simulink model "NonLinearControl"  (R2021b)
settings: Solver=VariableStepAuto  StartTime=0  StopTime=500  RelTol=1e-3
values from neighbouring files (symbols this model uses):
  accelerationLimit = 0.37    [ltdSimulationParameters.m]
  ageTrain = 0.85    [ltdSimulationParameters.m]
  decelerationLimit = 1.18    [ltdSimulationParameters.m]
  K = place(A,B,pole)    [ltdSimulationParameters.m]
  Ka = 0.07    [ltdSimulationParameters.m]
  M = 54.5    [ltdSimulationParameters.m]
  m = M * 10^3 + (load * weight)    (= 58980)    [ltdSimulationParameters.m]
  nP = 6    [ltdSimulationParameters.m]
  speedLimit = 55.88    [ltdSimulationParameters.m]
  theta = 4e-4    (= 0.0004)    [ltdSimulationParameters.m]
  wP = m/nP    (= 9830)    [ltdSimulationParameters.m]
  x_1 = 0    [ltdSimulationParameters.m]
  x_2 = 0    [ltdSimulationParameters.m]
undefined symbols (not defined in the file or in its folder): displaceRequired, magnitude
settings Model: SimulationMode=rapid-accelerator  Creator=User  LastModifiedBy=User
settings SolverCC: AlgebraicLoopSolver=TrustRegion
settings DebuggingCC: SFMachineParentedDataDiag=warning

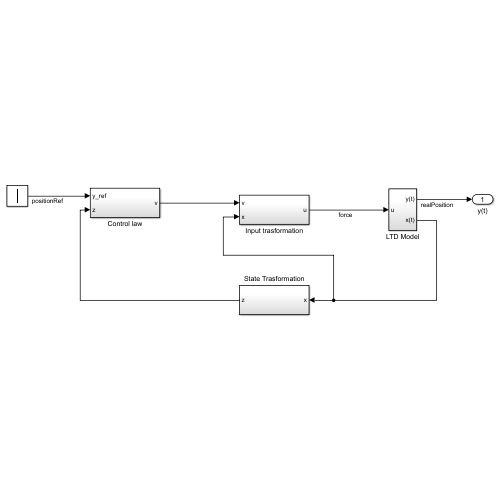
[thumbnail: Simulink's stored preview of the top-level diagram]
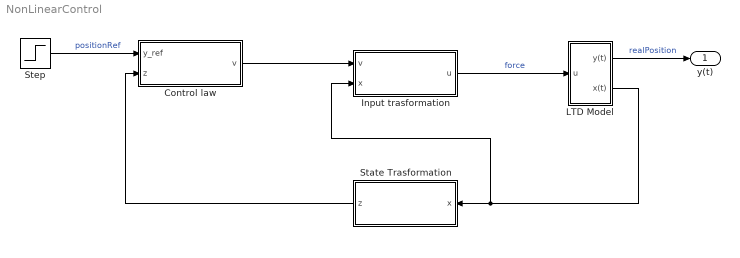
== system NonLinearControl ==
  Control law : Subsystem
  Input trasformation : Subsystem
  LTD Model : Subsystem
  State Trasformation : Subsystem
  Step : Step  After=displaceRequired  SampleTime=0
  y(t) : Outport
  wires:
  Input trasformation/1(u) -> LTD Model/1(u)  "force"
  LTD Model/2(x(t)) -> State Trasformation/1(x), Input trasformation/2(x)
  LTD Model/1(y(t)) -> y(t)/1  "realPosition"
  State Trasformation/1(z) -> Control law/2(z)
  Control law/1(v) -> Input trasformation/1(v)
  Step/1 -> Control law/1(y_ref)  "positionRef"

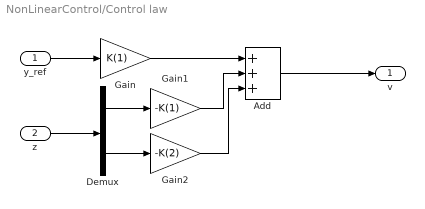
== system NonLinearControl/Control law ==
  y_ref : Inport
  z : Inport  Port=2
  Add : Sum  Inputs=+++
  Demux : Demux  Outputs=2
  Gain : Gain  Gain=K(1)
  Gain1 : Gain  Gain=-K(1)
  Gain2 : Gain  Gain=-K(2)
  v : Outport
  wires:
  z/1 -> Demux/1
  y_ref/1 -> Gain/1
  Gain/1 -> Add/1
  Demux/1 -> Gain1/1
  Demux/2 -> Gain2/1
  Gain1/1 -> Add/2
  Gain2/1 -> Add/3
  Add/1 -> v/1

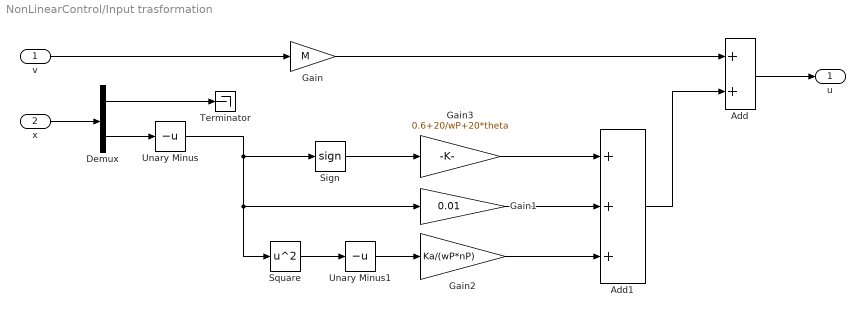
== system NonLinearControl/Input trasformation ==
  v : Inport
  x : Inport  Port=2
  Add : Sum
  Add1 : Sum  Inputs=+++
  Demux : Demux  Outputs=2
  Gain : Gain  Gain=M
  Gain1 : Gain  Gain=0.01
  Gain2 : Gain  Gain=Ka/(wP*nP)
  Gain3 : Gain  Gain=0.6+20/wP+20*theta
  Sign : Signum
  Square : Math  Operator=square  SaturateOnIntegerOverflow=on
  Terminator : Terminator
  Unary Minus : UnaryMinus
  Unary Minus1 : UnaryMinus
  u : Outport
  wires:
  v/1 -> Gain/1
  Gain/1 -> Add/1
  x/1 -> Demux/1
  Demux/1 -> Terminator/1
  Gain1/1 -> Add1/2
  Gain2/1 -> Add1/3
  Add1/1 -> Add/2
  Add/1 -> u/1
  Unary Minus1/1 -> Gain2/1
  Square/1 -> Unary Minus1/1
  Demux/2 -> Unary Minus/1
  Unary Minus/1 -> Sign/1, Gain1/1, Square/1
  Gain3/1 -> Add1/1
  Sign/1 -> Gain3/1

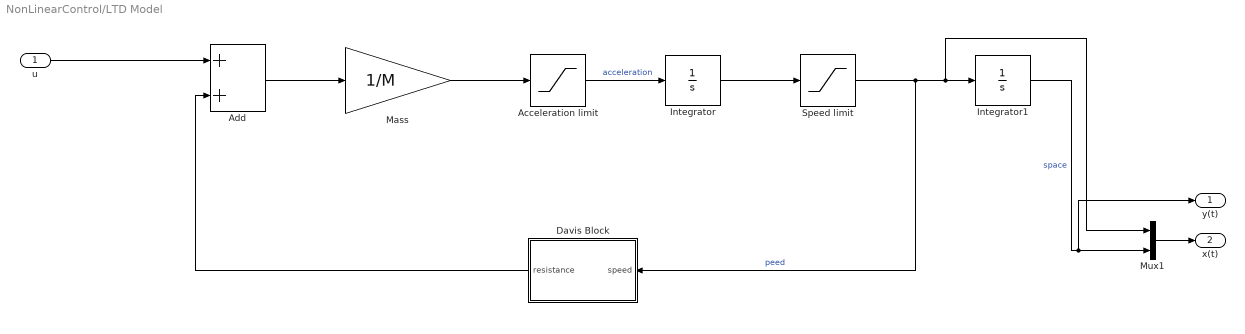
== system NonLinearControl/LTD Model ==
  u : Inport
  Acceleration limit : Saturate  UpperLimit=accelerationLimit  LowerLimit=-decelerationLimit
  Add : Sum
  Davis Block : Subsystem
  Integrator : Integrator  InitialCondition=x_2
  Integrator1 : Integrator  InitialCondition=x_1
  Mass : Gain  Gain=1/M
  Mux1 : Mux  Inputs=2
  Speed limit : Saturate  UpperLimit=speedLimit  LowerLimit=-speedLimit
  y(t) : Outport
  x(t) : Outport  Port=2
  wires:
  Acceleration limit/1 -> Integrator/1  "acceleration"
  Mass/1 -> Acceleration limit/1
  Speed limit/1 -> Davis Block/1(speed), Mux1/1, Integrator1/1  "peed"
  Integrator1/1 -> Mux1/2, y(t)/1  "space"
  Mux1/1 -> x(t)/1
  Integrator/1 -> Speed limit/1
  Add/1 -> Mass/1
  u/1 -> Add/1
  Davis Block/1(resistance) -> Add/2

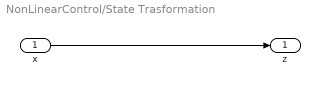
== system NonLinearControl/State Trasformation ==
  x : Inport
  z : Outport
  wires:
  x/1 -> z/1

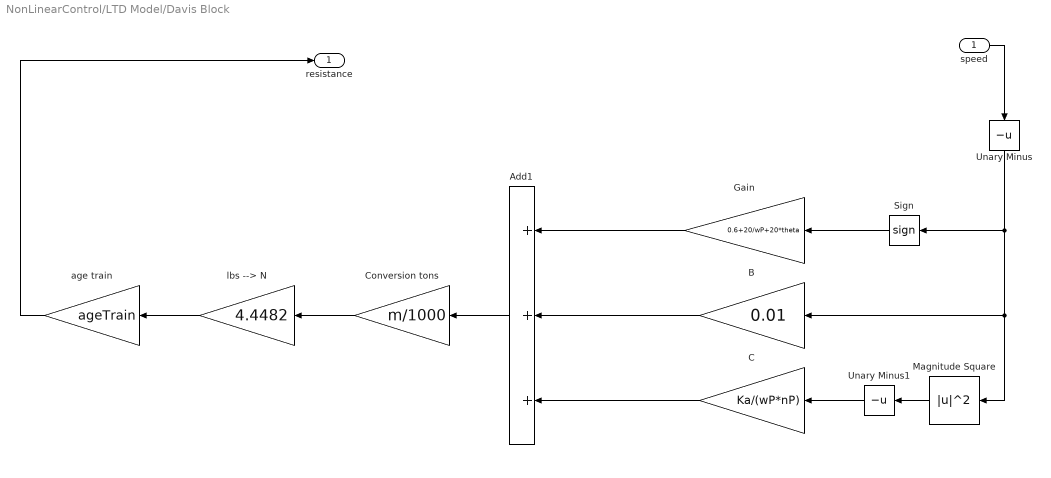
== system NonLinearControl/LTD Model/Davis Block ==
  speed : Inport
  Add1 : Sum  Inputs=+++
  B : Gain  Gain=0.01
  C : Gain  Gain=Ka/(wP*nP)
  Conversion tons : Gain  Gain=m/1000
  Gain : Gain  Gain=0.6+20/wP+20*theta
  Magnitude Square : Math  Operator=magnitude^2  SignedPower=on  RndMeth=Zero  SaturateOnIntegerOverflow=on
  Sign : Signum
  Unary Minus : UnaryMinus
  Unary Minus1 : UnaryMinus
  age train : Gain  Gain=ageTrain
  lbs --> N : Gain  Gain=4.4482
  resistance : Outport
  wires:
  lbs --> N/1 -> age train/1
  Unary Minus/1 -> Magnitude Square/1, B/1, Sign/1
  Gain/1 -> Add1/1
  Magnitude Square/1 -> Unary Minus1/1
  Conversion tons/1 -> lbs --> N/1
  Add1/1 -> Conversion tons/1
  B/1 -> Add1/2
  C/1 -> Add1/3
  Unary Minus1/1 -> C/1
  speed/1 -> Unary Minus/1
  Sign/1 -> Gain/1
  age train/1 -> resistance/1
